simulink model "singleCellElectricalModel"  (R2025a)
settings: Solver=ode15s  StartTime=0  StopTime=100000  MaxStep=1  RelTol=1e-5  AbsTol=1e-6
libraries: fl_lib x2, nesl_utility x2, batt_lib x1, Batteries_lib x1
settings Model: Creator=jagmohanfanshal  LastModifiedBy=jagmohanfanshal
settings SimscapeCC: SimscapeLogType=all

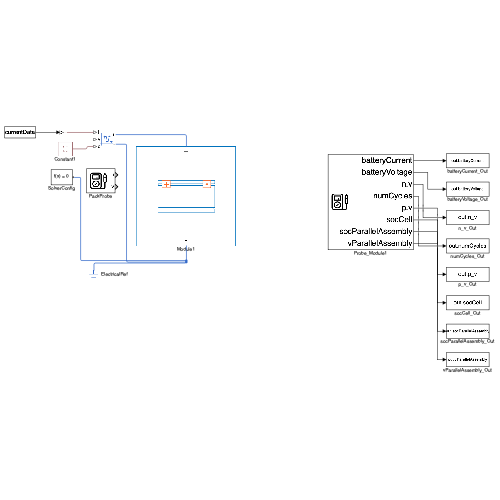
[thumbnail: Simulink's stored preview of the top-level diagram]
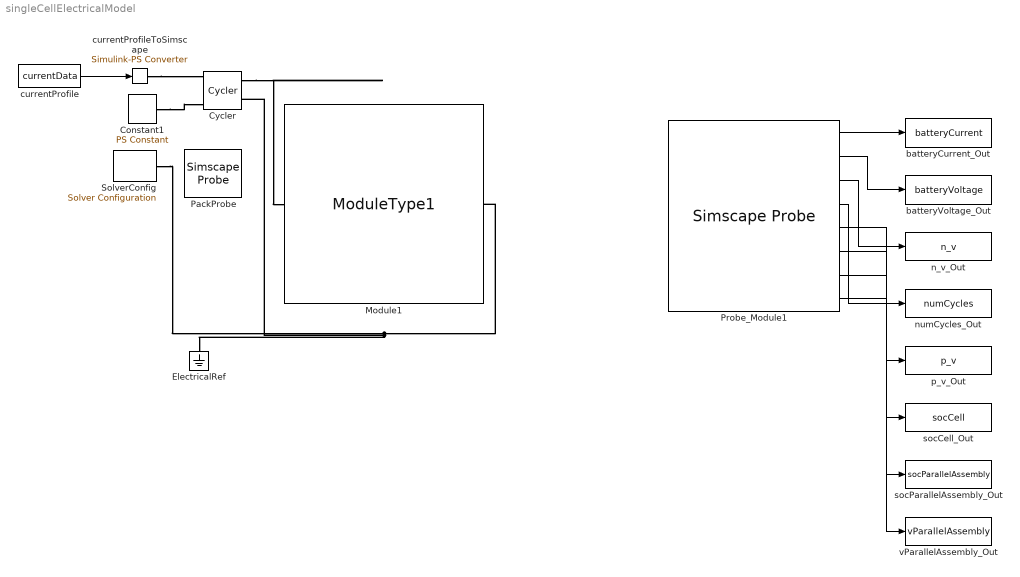
== system singleCellElectricalModel ==
  Constant1 : fl_lib/Physical Signals/Sources/PS Constant  constant=1
  Cycler : batt_lib/Cyclers/Cycler  current_option=simscape.battery.enum.cyclers.positive_current.Discharge  configuration_option=simscape.battery.enum.cyclers.device_configuration.Cycler
      settings: InternalSimscapePortConfiguration="{\"Bottom\":[],\"Left\":[{\"id\":\"iT\",\"label\":\"i\",\"type\":\"input\"},{\"id\":\"vT\",\"label\":\"v\",\"type\":\"input\"},{\"id\":\"c\",\"label\":\"c\",\"type\":\"input\"}],\"Right\":[{\"id\":\"p\",\"label\":\"+\",\"type\":\"foundation.electrical.electrical\"},{\"id\":\"n\",\"label\":\"-\",\"type\":\"foundation.electrical.electrical\"}],\"Top\":[]}"
  ElectricalRef : fl_lib/Electrical/Electrical Elements/Electrical Reference
  Module1 : Batteries_lib/Modules/ModuleType1  BatteryCapacityCell=Module1.BatteryCapacityCell A*hr  ExtrapolationMethodCell=simscape.enum.extrapolation.nearest  SOCBreakpointsCell=Module1.SOCBreakpointsCell  TemperatureBreakpointsCell=Module1.TemperatureBreakpointsCell K  OpenCircuitVoltageThermalCell=Module1.OpenCircuitVoltageThermalCell V  VoltageRangeCell=Module1.VoltageRangeCell V  ResistanceSOCBreakpointsCell=Module1.ResistanceSOCBreakpointsCell  ResistanceTemperatureBreakpointsCell=Module1.ResistanceTemperatureBreakpointsCell K  R0ThermalCell=Module1.R0ThermalCell Ohm  R1ThermalCell=Module1.R1ThermalCell Ohm  Tau1ThermalCell=Module1.Tau1ThermalCell s  SimulationTemperatureCell=Module1.batteryTemperature K  P=1  S=1  socCell_specify=on  socCell_priority=High  socCell=Module1.socCell  socCell_nominal_specify=off  socCell_nominal_value=1  socCell_nominal_unit=1  batteryVoltage_specify=on  batteryVoltage_priority=None  batteryVoltage=Module1.batteryVoltage V  batteryVoltage_nominal_specify=off  batteryVoltage_nominal_value=1  batteryVoltage_nominal_unit=V  batteryCurrent_specify=on  batteryCurrent_priority=None  batteryCurrent=Module1.batteryCurrent A  batteryCurrent_nominal_specify=off  batteryCurrent_nominal_value=1  batteryCurrent_nominal_unit=A  numCycles_specify=on  numCycles_priority=None  numCycles=Module1.numCycles  numCycles_nominal_specify=off  numCycles_nominal_value=1  numCycles_nominal_unit=1  vParallelAssembly_specify=on  vParallelAssembly_priority=None  vParallelAssembly=Module1.vParallelAssembly V  vParallelAssembly_nominal_specify=off  vParallelAssembly_nominal_value=1  vParallelAssembly_nominal_unit=V  socParallelAssembly_specify=on  socParallelAssembly_priority=None  socParallelAssembly=Module1.socParallelAssembly  socParallelAssembly_nominal_specify=off  socParallelAssembly_nominal_value=1  socParallelAssembly_nominal_unit=1
      settings: InternalSimscapePortConfiguration="{\"Bottom\":[{\"id\":\"n\",\"label\":\"-\",\"type\":\"foundation.electrical.electrical\"}],\"Left\":[],\"Right\":[],\"Top\":[{\"id\":\"p\",\"label\":\"+\",\"type\":\"foundation.electrical.electrical\"}]}"
  PackProbe : SimscapeProbe  BoundBlock=3  Variables="{\"i\":{\"Probing\":\"ON\"},\"v\":{\"Probing\":\"ON\"}}"
  Probe_Module1 : SimscapeProbe  BoundBlock=1  Variables="{\"batteryCurrent\":{\"Probing\":\"ON\"},\"batteryVoltage\":{\"Probing\":\"ON\"},\"n.v\":{\"Probing\":\"ON\"},\"numCycles\":{\"Probing\":\"ON\"},\"p.v\":{\"Probing\":\"ON\"},\"socCell\":{\"Probing\":\"ON\"},\"socParallelAssembly\":{\"Probing\":\"ON\"},\"vParallelAssembly\":{\"Probing\":\"ON\"}}"
  SolverConfig : nesl_utility/Solver Configuration  PhysicalDomain=network_engine_domain  SubClassName=solver  LeftPortType=input  RightPortType=generic  Tones=[]  Harmonics=[]  SimulateNoise=off  Profile=off  UseLocalSampling=off  EnableSwitchedLinearOptims=on  FrequencyDomain=off  UseCCode=off  RelTol=0.001  AbsTol=0.001  MinStep=1e-09  ToWorkspace=off  RevertToSquareIcSolve=off  NumHomotopyIterations=100  PhasorMode=off  PhasorModeNumHarmonics=1  ConsistencySolver=NEWTON_XTOL_AFTER_FTOL  IndexReductionMethod=DerivativeReplacement  DoDC=off  ResidualTolerance=1e-09  ConsistencyTolSource=GLOBAL  ConsistencyAbsTol=0.001  ConsistencyRelTol=0.001  ConsistencyTolFactor=0.001  UseLocalSolver=off  LocalSolverChoice=NE_BACKWARD_EULER_ADVANCER  ResolveIndetEquations=on  FunctionEvalNumThread=1  LocalSolverSampleTime=0.001  DoFixedCost=off  MaxNonlinIter=3  MaxModeIter=2  ComputeImpulses=off  ImpulseIterations=2  LinearAlgebra=auto  LinearAlgebraNumThread=0  EquationFormulation=NE_TIME_EF  DelaysMemoryBudget=1024  AutomaticFiltering=on  FilteringTimeConstant=0.001  PartitionStorageMethod=AS_NEEDED  PartitionMemoryBudget=1024  PartitionMethod=ROBUST  MultibodyUseLocalSolver=off  MultibodyLocalSolverChoice=ODE1  MultibodyLocalSolverSampleTime=0.001
  batteryCurrent_Out : ToWorkspace  VariableName=batteryCurrent  SaveFormat=Structure With Time  SampleTime=-1
  batteryVoltage_Out : ToWorkspace  VariableName=batteryVoltage  SaveFormat=Structure With Time  SampleTime=-1
  currentProfile : FromWorkspace  VariableName=currentData  SampleTime=10
  currentProfileToSimscape : nesl_utility/Simulink-PS Converter  PhysicalDomain=network_engine_domain  SubClassName=ps_input  LeftPortType=input  RightPortType=output  PseudoPeriodic=off  Frequencies=[]  NoiseDistribution=none  NoiseParameters=[]  Unit=1  AffineConversion=off  FilteringAndDerivatives=provide  SimscapeFilterOrder=1  InputFilterTimeConstant=0.001  UdotUserProvided=0
  n_v_Out : ToWorkspace  VariableName=n_v  SaveFormat=Structure With Time  SampleTime=-1
  numCycles_Out : ToWorkspace  VariableName=numCycles  SaveFormat=Structure With Time  SampleTime=-1
  p_v_Out : ToWorkspace  VariableName=p_v  SaveFormat=Structure With Time  SampleTime=-1
  socCell_Out : ToWorkspace  VariableName=socCell  SaveFormat=Structure With Time  SampleTime=-1
  socParallelAssembly_Out : ToWorkspace  VariableName=socParallelAssembly  SaveFormat=Structure With Time  SampleTime=-1
  vParallelAssembly_Out : ToWorkspace  VariableName=vParallelAssembly  SaveFormat=Structure With Time  SampleTime=-1
  wires:
  currentProfile/1 -> currentProfileToSimscape/1
  Probe_Module1/1 -> batteryCurrent_Out/1
  Probe_Module1/2 -> batteryVoltage_Out/1
  Probe_Module1/3 -> n_v_Out/1
  Probe_Module1/4 -> numCycles_Out/1
  Probe_Module1/5 -> p_v_Out/1
  Probe_Module1/6 -> socCell_Out/1
  Probe_Module1/7 -> socParallelAssembly_Out/1
  Probe_Module1/8 -> vParallelAssembly_Out/1
  connections:
  Cycler/RConn1 -- Module1/LConn1
  SolverConfig/RConn1 -- Cycler/RConn2 -- ElectricalRef/LConn1 -- Module1/RConn1
  Constant1/RConn1 -- Cycler/LConn3
  currentProfileToSimscape/RConn1 -- Cycler/LConn1
